simulink model "SHEV_EXAMPLE1"  (R2024a)
settings: Solver=VariableStepAuto  StartTime=0  StopTime=40  RelTol=1e-3
model workspace (MAT data in the model file):
  rpm0 = Simulink.Parameter
  rpm0.Value = 2000
  rpm0.Complexity = 'real'
  rpm0.Dimensions = [1 1]
  rpm0.DataType = 'double'
  v0 = Simulink.Parameter
  v0.Value = 15
  v0.Complexity = 'real'
  v0.Dimensions = [1 1]
  v0.DataType = 'double'
  wheel_radius = Simulink.Parameter
  wheel_radius.Value = 0.3
  wheel_radius.Complexity = 'real'
  wheel_radius.Dimensions = [1 1]
  wheel_radius.DataType = 'double'
libraries: fl_lib x27, nesl_utility x16, sdl_lib x8, autolibshared x2, ee_lib x1
settings Model: Creator=DELL  LastModifiedBy=DELL

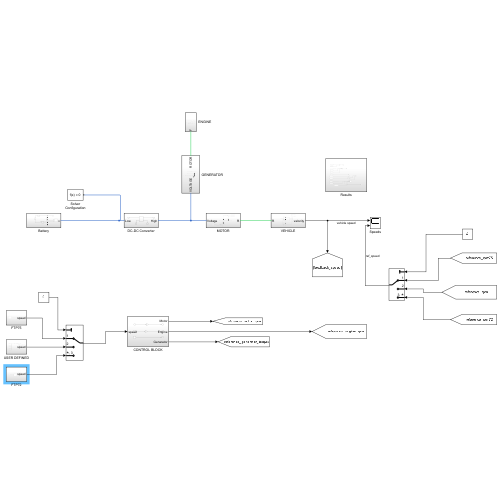
[thumbnail: Simulink's stored preview of the top-level diagram]
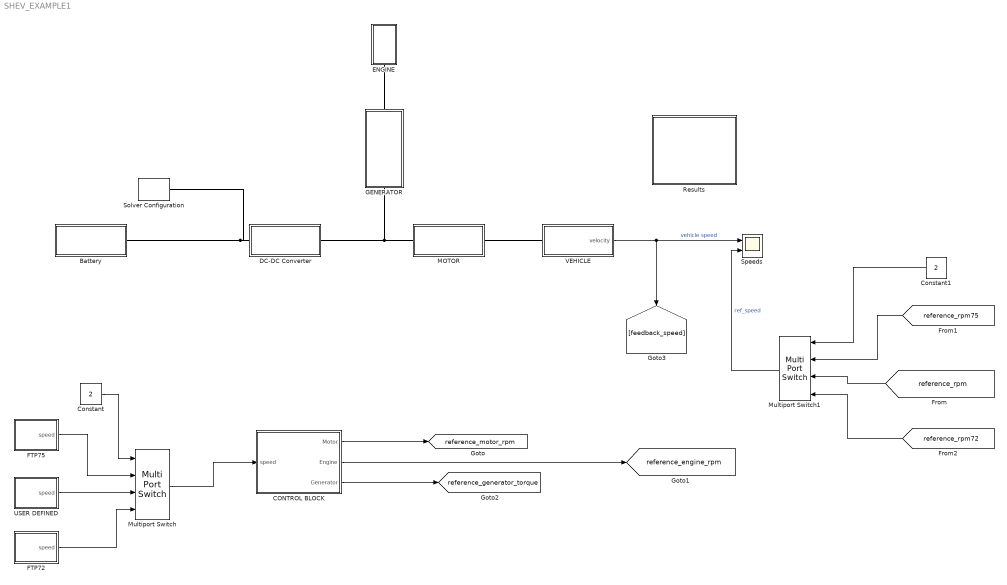
== system SHEV_EXAMPLE1 ==
  Battery : Subsystem
  CONTROL BLOCK : Subsystem
  Constant : Constant  Value=2
  Constant1 : Constant  Value=2
  DC-DC Converter : Subsystem
  ENGINE : Subsystem
  FTP72 : Subsystem
  FTP75 : Subsystem
  GENERATOR : Subsystem
  MOTOR : Subsystem
  Multiport Switch : MultiPortSwitch  SaturateOnIntegerOverflow=off  InputSameDT=off
  Multiport Switch1 : MultiPortSwitch  SaturateOnIntegerOverflow=off  InputSameDT=off
  Results : Subsystem
  Solver Configuration : nesl_utility/Solver Configuration  PhysicalDomain=network_engine_domain  SubClassName=solver  LeftPortType=input  RightPortType=generic  Tones=[]  Harmonics=[]  SimulateNoise=off  Profile=off  UseLocalSampling=off  EnableSwitchedLinearOptims=on  FrequencyDomain=off  UseCCode=off  RelTol=0.001  AbsTol=0.001  MinStep=1e-09  ToWorkspace=off  RevertToSquareIcSolve=off  NumHomotopyIterations=100  PhasorMode=off  PhasorModeNumHarmonics=1  ConsistencySolver=NEWTON_XTOL_AFTER_FTOL  IndexReductionMethod=DerivativeReplacement  DoDC=off  ResidualTolerance=1e-09  ConsistencyTolSource=GLOBAL  ConsistencyAbsTol=0.001  ConsistencyRelTol=0.001  ConsistencyTolFactor=0.001  UseLocalSolver=off  LocalSolverChoice=NE_BACKWARD_EULER_ADVANCER  ResolveIndetEquations=on  FunctionEvalNumThread=1  LocalSolverSampleTime=0.001  DoFixedCost=off  MaxNonlinIter=3  MaxModeIter=2  ComputeImpulses=off  ImpulseIterations=2  LinearAlgebra=auto  LinearAlgebraNumThread=0  EquationFormulation=NE_TIME_EF  DelaysMemoryBudget=1024  AutomaticFiltering=on  FilteringTimeConstant=0.001  PartitionStorageMethod=AS_NEEDED  PartitionMemoryBudget=1024  PartitionMethod=ROBUST  MultibodyUseLocalSolver=off  MultibodyLocalSolverChoice=ODE1  MultibodyLocalSolverSampleTime=0.001
  Speeds : Scope  NumInputPorts=2
  USER DEFINED : Subsystem
  VEHICLE : Subsystem
  tag scope: reference_engine_rpm=global, reference_generator_torque=global, reference_motor_rpm=global
  wires:
  [reference_rpm] -> Multiport Switch1/3
  CONTROL BLOCK/1(Motor) -> [reference_motor_rpm]
  VEHICLE/1(velocity) -> [feedback_speed], Speeds/1  "vehicle speed"
  CONTROL BLOCK/3(Generator) -> [reference_generator_torque]
  CONTROL BLOCK/2(Engine) -> [reference_engine_rpm]
  Constant/1 -> Multiport Switch/1
  FTP75/1(speed) -> Multiport Switch/2
  USER DEFINED/1(speed) -> Multiport Switch/3
  FTP72/1(speed) -> Multiport Switch/4
  Multiport Switch/1 -> CONTROL BLOCK/1(speed)
  Constant1/1 -> Multiport Switch1/1
  [reference_rpm75] -> Multiport Switch1/2
  [reference_rpm72] -> Multiport Switch1/4
  Multiport Switch1/1 -> Speeds/2  "ref_speed"
  connections:
  DC-DC Converter/LConn1 -- Solver Configuration/RConn1 -- Battery/RConn1
  MOTOR/RConn1 -- VEHICLE/LConn1
  ENGINE/LConn1 -- GENERATOR/RConn1
  DC-DC Converter/RConn1 -- GENERATOR/LConn1 -- MOTOR/LConn1

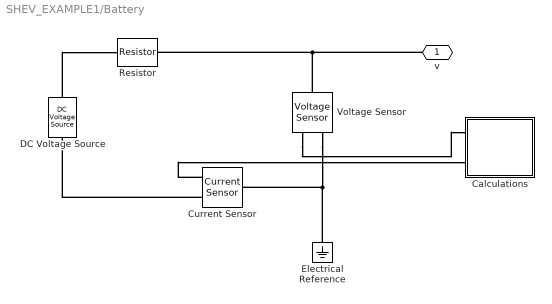
== system SHEV_EXAMPLE1/Battery ==
  Calculations : Subsystem
  Current Sensor : fl_lib/Electrical/Electrical Sensors/Current Sensor
  DC Voltage Source : ee_lib/Additional Components/SPICE Sources/DC Voltage Source  DC=200 V
  Electrical Reference : fl_lib/Electrical/Electrical Elements/Electrical Reference
  Resistor : fl_lib/Electrical/Electrical Elements/Resistor  R=0.05 Ohm  i_specify=off  i_priority=None  i=0 A  i_nominal_specify=off  i_nominal_value=1  i_nominal_unit=A  v_specify=off  v_priority=None  v=0 V  v_nominal_specify=off  v_nominal_value=1  v_nominal_unit=V
  Voltage Sensor : fl_lib/Electrical/Electrical Sensors/Voltage Sensor
  v : PMIOPort  Side=Right
  connections:
  DC Voltage Source/LConn1 -- Resistor/LConn1
  Current Sensor/RConn2 -- DC Voltage Source/RConn1
  Voltage Sensor/LConn1 -- Resistor/RConn1 -- v/RConn1
  Voltage Sensor/RConn2 -- Current Sensor/LConn1 -- Electrical Reference/LConn1
  Voltage Sensor/RConn1 -- Calculations/RConn1
  Current Sensor/RConn1 -- Calculations/RConn2

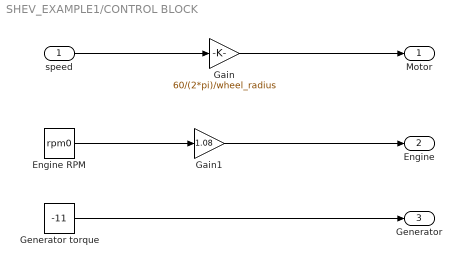
== system SHEV_EXAMPLE1/CONTROL BLOCK ==
  speed : Inport
  Engine RPM : Constant  Value=rpm0
  Gain : Gain  Gain=60/(2*pi)/wheel_radius
  Gain1 : Gain  Gain=1.08
  "Generator torque " : Constant  Value=-11
  Motor : Outport
  Engine : Outport  Port=2
  Generator : Outport  Port=3
  wires:
  speed/1 -> Gain/1
  Gain/1 -> Motor/1
  Engine RPM/1 -> Gain1/1
  Gain1/1 -> Engine/1
  "Generator torque "/1 -> Generator/1

== system SHEV_EXAMPLE1/DC-DC Converter ==
  Electrical Reference : fl_lib/Electrical/Electrical Elements/Electrical Reference
  Electrical Reference1 : fl_lib/Electrical/Electrical Elements/Electrical Reference
  Ideal Transformer : fl_lib/Electrical/Electrical Elements/Ideal Transformer  n=200/500  i1_specify=off  i1_priority=None  i1=0 A  i1_nominal_specify=off  i1_nominal_value=1  i1_nominal_unit=A  v1_specify=off  v1_priority=None  v1=0 V  v1_nominal_specify=off  v1_nominal_value=1  v1_nominal_unit=V  i2_specify=off  i2_priority=None  i2=0 A  i2_nominal_specify=off  i2_nominal_value=1  i2_nominal_unit=A  v2_specify=off  v2_priority=None  v2=0 V  v2_nominal_specify=off  v2_nominal_value=1  v2_nominal_unit=V
  Low : PMIOPort  Side=Left
  High : PMIOPort  Port=2  Side=Right
  connections:
  Ideal Transformer/LConn2 -- Electrical Reference/LConn1
  Ideal Transformer/RConn2 -- Electrical Reference1/LConn1
  Low/RConn1 -- Ideal Transformer/LConn1
  High/RConn1 -- Ideal Transformer/RConn1

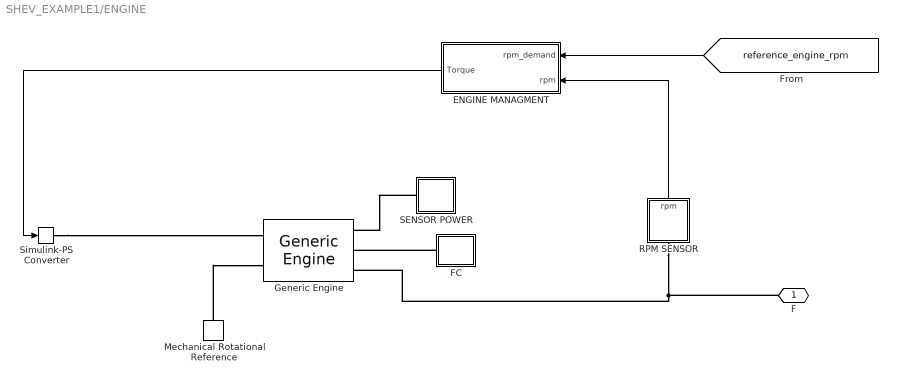
== system SHEV_EXAMPLE1/ENGINE ==
  ENGINE MANAGMENT : Subsystem
  FC : Subsystem
  Generic Engine : sdl_lib/Engines & Motors/Generic Engine  input_type=sdl.enum.GenericEngineInputType.NormalizedThrottle  model_parameterization=sdl.enum.engineParameterization.polynomial  engine_type=sdl.enum.engineType.SI  Trq_max=380 N*m  w_Trq_max=4300 rpm  P_max=50e3 W  w_P_max=5500 rpm  w_max=7000 rpm  w_min=500 rpm  w_tab=[500, 1000, 2000, 3000, 4300, 5000, 6000, 7000] rpm  trq_tab=[250, 280, 330, 360, 380, 370, 350, 310] N*m  pwr_tab=[10, 30, 70, 110, 165, 190, 220, 230] kW  interp_method=simscape.enum.interpolation.linear  w_thr=20 rpm  model_inertia=sdl.enum.model_inertia.on  inertia=0.2 kg*m^2  initial_velocity=rpm0 rpm  model_time_constant=sdl.enum.lagOffOn.on  time_constant=0.2 s  initial_normalized_throttle=0  fc_model=sdl.enum.fuel_consumption_model.BSFCSpeedBMEP  fc_per_rev=25 mg/rev  fc_w_tab=[ 1000 2e+3 3e+3 4e+3 5e+3 6e+3 ] rpm  fc_trq_tab=[0, 80, 160, 200, 240, 320, 360, 400] N*m  fc_tab=[.5, .9, 1.4, 1.6, 1.9, 2.7, 3.4, 4.4; 1, 1.7, 2.7, 3.1, 3.6, 5, 6, 7.4; 1.4, 2.7, 4, 4.8, 5.6, 7.5, 8.5, 10.5; 2, 3.6, 5.8, 6.7, 8, 10.4, 11.7, 13.3; 2.5, 4.8, 7.9, 9.4, 10.8, 14, 16.2, 18.6; 3.1, 6, 10.3, 11.9, 13.8, 18.4, 22, 26.5] g/s  bmep_tab=[ 0 250 500 625 750 1000 1.15e+3 1.25e+3 ] kPa  bsfc_tab=[ 410 380 300 280 270 290 320 380; 410 370 290 270 260 270 285 320; 415 380 290 275 265 270 270 300; 420 390 310 290 285 280 280 285; 430 410 340 320 310 300 310 320; 450 430 370 340 330 330 350 380 ] g/hr/kW  fc_interp_method=simscape.enum.interpolation.linear  displaced_volume=400 cm^3  rev_per_cycle=2  idle_speed=false  idle_speed_reference=1000 rpm  tau_controller=1 s  idle_w_thr=1 rpm  redline=false  redline_speed=5000 rpm  tau_redline=1 s  redline_w_thr=1 rpm
      settings: InternalSimscapePortConfiguration="{\"Bottom\":[],\"Left\":[{\"id\":\"ThrNorm\",\"label\":\"Thr\",\"type\":\"input\"},{\"id\":\"B\",\"label\":\"B\",\"type\":\"foundation.mechanical.rotational.rotational\"}],\"Right\":[{\"id\":\"P\",\"label\":\"P\",\"type\":\"output\"},{\"id\":\"FC\",\"label\":\"FC\",\"type\":\"output\"},{\"id\":\"F\",\"label\":\"F\",\"type\":\"foundation.mechanical.rotational.rotational\"}],\"Top\":[]}"
  Mechanical Rotational Reference : fl_lib/Mechanical/Rotational Elements/Mechanical Rotational Reference
  RPM SENSOR : Subsystem
  SENSOR POWER : Subsystem
  Simulink-PS Converter : nesl_utility/Simulink-PS Converter  PhysicalDomain=network_engine_domain  SubClassName=ps_input  LeftPortType=input  RightPortType=output  PseudoPeriodic=off  Frequencies=[]  NoiseDistribution=none  NoiseParameters=[]  Unit=1  AffineConversion=off  FilteringAndDerivatives=zero  SimscapeFilterOrder=1  InputFilterTimeConstant=0.001  UdotUserProvided=0
  F : PMIOPort  Side=Left
  wires:
  [reference_engine_rpm] -> ENGINE MANAGMENT/1(rpm_demand)
  RPM SENSOR/1(rpm) -> ENGINE MANAGMENT/2(rpm)
  ENGINE MANAGMENT/1(Torque) -> Simulink-PS Converter/1
  connections:
  Mechanical Rotational Reference/LConn1 -- Generic Engine/LConn2
  Simulink-PS Converter/RConn1 -- Generic Engine/LConn1
  SENSOR POWER/LConn1 -- Generic Engine/RConn1
  FC/LConn1 -- Generic Engine/RConn2
  RPM SENSOR/LConn1 -- F/RConn1 -- Generic Engine/RConn3

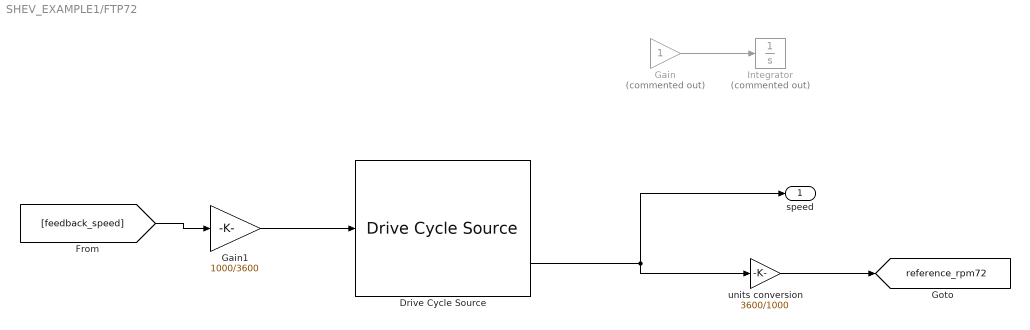
== system SHEV_EXAMPLE1/FTP72 ==
  Drive Cycle Source : autolibshared/Drive Cycle Source  cycleVar=FTP72  fileVar=cycleFTP75.mat  tfinal="1372  seconds"  cycleRepeat=off  outAccPort=off  outGearPort=off  gearList=No gear data  t_wot1=5  xdot_woto=0  xdot_wot1=30  t_wot2=20  xdot_wot2=0  t_wotend=30  srcUnit=m/s  outUnit=m/s  srcAccUnit=m/s/s  outAccUnit=m/s^2  dt=0  aMode=1  faultOption=on  velBnd=2  velBndUnit=mph  inUnit=m/s  timeBnd=1  failOption=off  stopSim=off  maxFaultCnt=10  maxFaultTime=2  maxTotFaultTime=15  traceOption=off  dtTrace=1  traceWindow=10  lastDCname=FTP72  lastOutUnit=mph  lastDT=0  lastTB=1  lastSB=2  forceCalcBound=off
  Gain : Gain  Commented=on
  Gain1 : Gain  Gain=1000/3600
  Integrator : Integrator  Commented=on  InitialCondition=v0
  units conversion : Gain  Gain=3600/1000
  speed : Outport
  tag scope: reference_rpm72=global
  wires:
  Gain/1 -> Integrator/1
  units conversion/1 -> [reference_rpm72]
  Drive Cycle Source/2 -> speed/1, units conversion/1
  Gain1/1 -> Drive Cycle Source/1
  [feedback_speed] -> Gain1/1

== system SHEV_EXAMPLE1/FTP75 ==
  Drive Cycle Source : autolibshared/Drive Cycle Source  cycleVar=FTP75  fileVar=cycleFTP75.mat  tfinal="2474  seconds"  cycleRepeat=off  outAccPort=off  outGearPort=off  gearList=No gear data  t_wot1=5  xdot_woto=0  xdot_wot1=30  t_wot2=20  xdot_wot2=0  t_wotend=30  srcUnit=m/s  outUnit=m/s  srcAccUnit=m/s/s  outAccUnit=m/s^2  dt=0  aMode=1  faultOption=off  velBnd=2  velBndUnit=mph  inUnit=m/s  timeBnd=1  failOption=off  stopSim=off  maxFaultCnt=10  maxFaultTime=2  maxTotFaultTime=15  traceOption=off  dtTrace=1  traceWindow=10  lastDCname=FTP75  lastOutUnit=mph  lastDT=0  lastTB=1  lastSB=2  forceCalcBound=off
  units conversion : Gain  Gain=3600/1000
  speed : Outport
  tag scope: reference_rpm75=global
  wires:
  units conversion/1 -> [reference_rpm75]
  Drive Cycle Source/1 -> units conversion/1, speed/1

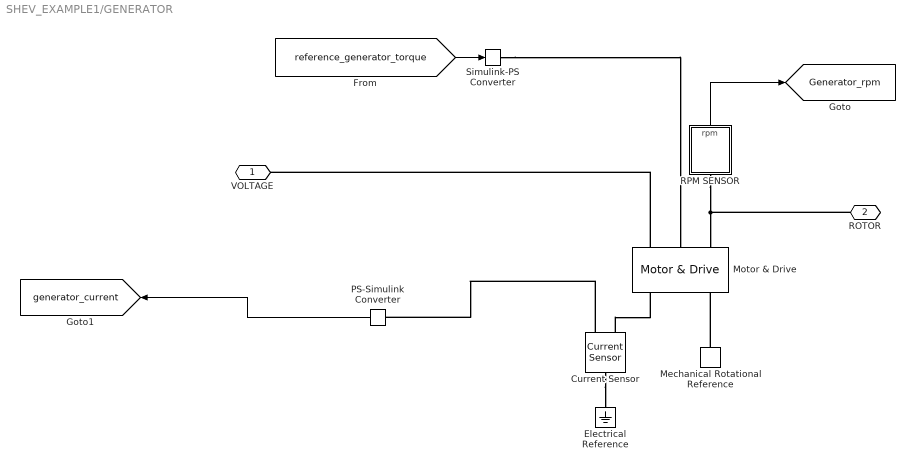
== system SHEV_EXAMPLE1/GENERATOR ==
  Current Sensor : fl_lib/Electrical/Electrical Sensors/Current Sensor
  Electrical Reference : fl_lib/Electrical/Electrical Elements/Electrical Reference
  Mechanical Rotational Reference : fl_lib/Mechanical/Rotational Elements/Mechanical Rotational Reference
  Motor & Drive : sdl_lib/Engines & Motors/Motor & Drive  torque_max=400 N*m  power_max=200 kW  Tc=0.2 s  eff=97  w_eff=600 rpm  T_eff=300 N*m  thermal_port=simscape.enum.thermaleffects.omit  thermal_mass=100 J/K  temperature_specify=off  temperature_priority=High  temperature=300 K  temperature_nominal_specify=off  temperature_nominal_value=1  temperature_nominal_unit=K
      settings: InternalSimscapePortConfiguration="{\"Bottom\":[],\"Left\":[{\"id\":\"Vp\",\"label\":\"+\",\"type\":\"foundation.electrical.electrical\"},{\"id\":\"Tr\",\"label\":\"Tr\",\"type\":\"input\"},{\"id\":\"R\",\"label\":\"R\",\"type\":\"foundation.mechanical.rotational.rotational\"}],\"Right\":[{\"id\":\"Vm\",\"label\":\"-\",\"type\":\"foundation.electrical.electrical\"},{\"id\":\"Omega\",\"label\":\"w\",\"type\":\"output\"},{\"id\":\"C\",\"label\":\"C\",\"type\":\"foundation.mechanical.rotational.rotational\"}],\"Top\":[]}"
  PS-Simulink Converter : nesl_utility/PS-Simulink Converter  PhysicalDomain=network_engine_domain  SubClassName=ps_output  LeftPortType=input  RightPortType=output  PseudoPeriodic=off  Frequencies=[]  VectorFormat=1-D array  Unit=A  AffineConversion=off
  RPM SENSOR : Subsystem
  Simulink-PS Converter : nesl_utility/Simulink-PS Converter  PhysicalDomain=network_engine_domain  SubClassName=ps_input  LeftPortType=input  RightPortType=output  PseudoPeriodic=off  Frequencies=[]  NoiseDistribution=none  NoiseParameters=[]  Unit=N*m  AffineConversion=off  FilteringAndDerivatives=zero  SimscapeFilterOrder=1  InputFilterTimeConstant=0.001  UdotUserProvided=0
  VOLTAGE : PMIOPort  Side=Left
  ROTOR : PMIOPort  Port=2  Side=Right
  tag scope: Generator_rpm=global, generator_current=global
  wires:
  [reference_generator_torque] -> Simulink-PS Converter/1
  RPM SENSOR/1(rpm) -> [Generator_rpm]
  PS-Simulink Converter/1 -> [generator_current]
  connections:
  RPM SENSOR/LConn1 -- Motor & Drive/LConn3 -- ROTOR/RConn1
  Simulink-PS Converter/RConn1 -- Motor & Drive/LConn2
  Mechanical Rotational Reference/LConn1 -- Motor & Drive/RConn3
  Current Sensor/RConn1 -- PS-Simulink Converter/LConn1
  Motor & Drive/LConn1 -- VOLTAGE/RConn1
  Current Sensor/LConn1 -- Electrical Reference/LConn1
  Current Sensor/RConn2 -- Motor & Drive/RConn1

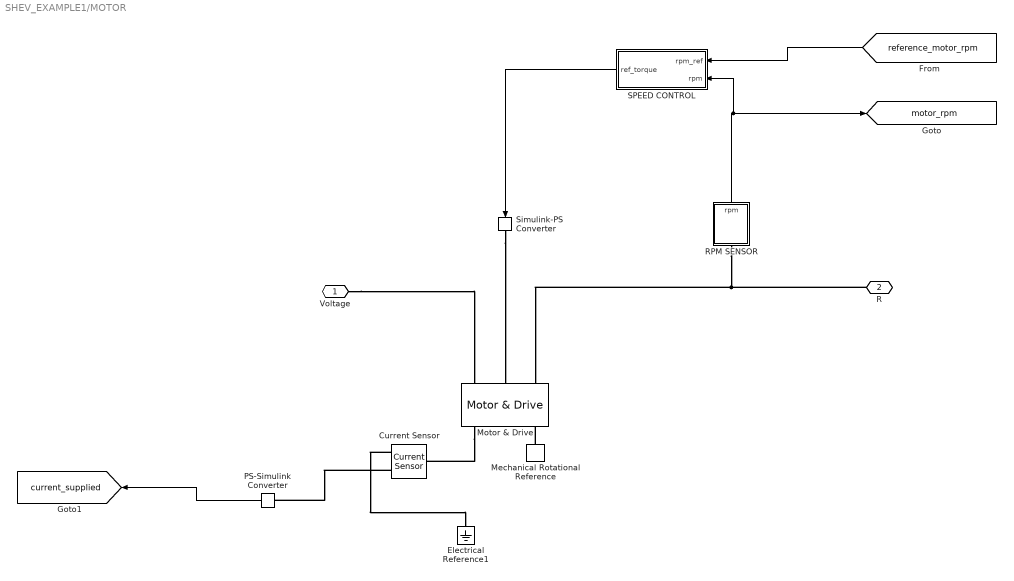
== system SHEV_EXAMPLE1/MOTOR ==
  Current Sensor : fl_lib/Electrical/Electrical Sensors/Current Sensor
  Electrical Reference1 : fl_lib/Electrical/Electrical Elements/Electrical Reference
  Mechanical Rotational Reference : fl_lib/Mechanical/Rotational Elements/Mechanical Rotational Reference
  Motor & Drive : sdl_lib/Engines & Motors/Motor & Drive  torque_max=400 N*m  power_max=200 kW  Tc=0.2 s  eff=97  w_eff=600 rpm  T_eff=300 N*m  thermal_port=simscape.enum.thermaleffects.omit  thermal_mass=100 J/K  temperature_specify=off  temperature_priority=High  temperature=300 K  temperature_nominal_specify=off  temperature_nominal_value=1  temperature_nominal_unit=K
      settings: InternalSimscapePortConfiguration="{\"Bottom\":[],\"Left\":[{\"id\":\"Vp\",\"label\":\"+\",\"type\":\"foundation.electrical.electrical\"},{\"id\":\"Tr\",\"label\":\"Tr\",\"type\":\"input\"},{\"id\":\"R\",\"label\":\"R\",\"type\":\"foundation.mechanical.rotational.rotational\"}],\"Right\":[{\"id\":\"Vm\",\"label\":\"-\",\"type\":\"foundation.electrical.electrical\"},{\"id\":\"Omega\",\"label\":\"w\",\"type\":\"output\"},{\"id\":\"C\",\"label\":\"C\",\"type\":\"foundation.mechanical.rotational.rotational\"}],\"Top\":[]}"
  PS-Simulink Converter : nesl_utility/PS-Simulink Converter  PhysicalDomain=network_engine_domain  SubClassName=ps_output  LeftPortType=input  RightPortType=output  PseudoPeriodic=off  Frequencies=[]  VectorFormat=1-D array  Unit=A  AffineConversion=off
  RPM SENSOR : Subsystem
  SPEED CONTROL : Subsystem
  Simulink-PS Converter : nesl_utility/Simulink-PS Converter  PhysicalDomain=network_engine_domain  SubClassName=ps_input  LeftPortType=input  RightPortType=output  PseudoPeriodic=off  Frequencies=[]  NoiseDistribution=none  NoiseParameters=[]  Unit=N*m  AffineConversion=off  FilteringAndDerivatives=zero  SimscapeFilterOrder=1  InputFilterTimeConstant=0.001  UdotUserProvided=0
  Voltage : PMIOPort  Side=Left
  R : PMIOPort  Port=2  Side=Right
  tag scope: current_supplied=global, motor_rpm=global
  wires:
  RPM SENSOR/1(rpm) -> SPEED CONTROL/2(rpm), [motor_rpm]
  SPEED CONTROL/1(ref_torque) -> Simulink-PS Converter/1
  [reference_motor_rpm] -> SPEED CONTROL/1(rpm_ref)
  PS-Simulink Converter/1 -> [current_supplied]
  connections:
  Voltage/RConn1 -- Motor & Drive/LConn1
  Mechanical Rotational Reference/LConn1 -- Motor & Drive/RConn3
  R/RConn1 -- RPM SENSOR/LConn1 -- Motor & Drive/LConn3
  Simulink-PS Converter/RConn1 -- Motor & Drive/LConn2
  Current Sensor/RConn1 -- PS-Simulink Converter/LConn1
  Motor & Drive/RConn1 -- Current Sensor/LConn1
  Current Sensor/RConn2 -- Electrical Reference1/LConn1

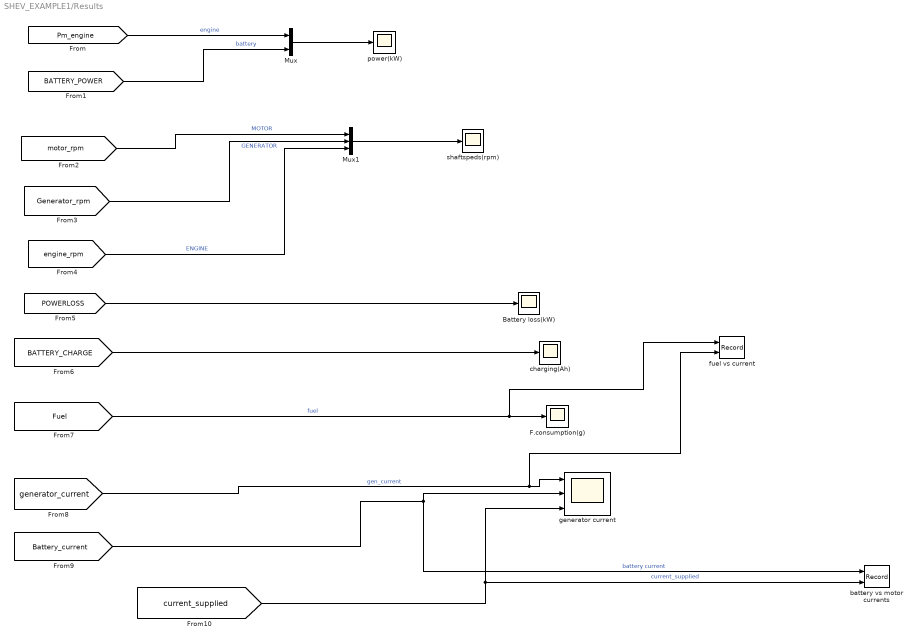
== system SHEV_EXAMPLE1/Results ==
  Battery loss(kW) : Scope
  F.consumption(g) : Scope
  Mux : Mux  Inputs=2
  Mux1 : Mux  Inputs=3
  battery vs motor currents : Record  FileSettingsInternal="{\"entries\":[{\"content\":{\"excelSettings\":{\"content\":{},\"type\":\"Streamout.ExcelSettings\"}},\"type\":\"Streamout.FileSettingStorage\",\"uuid\":\"\"}],\"packageUris\":[\"http:\\/\\/schema.mathworks.com\\/mf0\\/streamout_blocks\\/R2020a\"],\"version\":\"1.0\"}"  Layout=[1 1]  SignalsInternal="{\"entries\":[{\"content\":{\"signals\":[{\"content\":{\"blockPath\":[],\"dimensions\":[1],\"domain\":\"\",\"lineColor\":\"#0072bd\",\"lineWidth\":2,\"port\":1,\"sid\":[\"\"],\"signalID\":1,\"signalName\":\"battery current\"},\"type\":\"RecordBlkView.Signal\",\"uuid\":\"\"},{\"content\":{\"blockPath\":[],\"dimensions\":[1],\"domain\":\"\",\"lineColor\":\"#139fff\",\"plots\":[ 1 ],\"port\":2,\"sid\":[\"\"],\"signalID\":2,\"signalName\":\"current_supplied\"},\"type\":\"RecordBlkView.Signal\",\"uuid\":\"\"}]},\"type\":\"RecordBlkView.InputSignals\",\"uuid\":\"\"}],\"packageUris\":[\"http:\\/\\/schema.mathworks.com\\/mf0\\/streamout_blocks\\/R2020a\"],\"version\":\"1.0\"}"  VisualizationBindings="{\"xyplotplugin\":{\"info\":[{\"series\":[{\"bindingParametersList\":[{\"parameter\":\"Y-Axis\",\"signalID\":2,\"signalName\":\"current_supplied\"}],\"seriesID\":0}],\"subplotID\":1}]}}"  CompatibilityTag=XY
  charging(Ah) : Scope
  "fuel vs current " : Record  FileSettingsInternal="{\"entries\":[{\"content\":{\"excelSettings\":{\"content\":{},\"type\":\"Streamout.ExcelSettings\"}},\"type\":\"Streamout.FileSettingStorage\",\"uuid\":\"\"}],\"packageUris\":[\"http:\\/\\/schema.mathworks.com\\/mf0\\/streamout_blocks\\/R2020a\"],\"version\":\"1.0\"}"  Layout=[1 1]  SignalsInternal="{\"entries\":[{\"content\":{\"signals\":[{\"content\":{\"blockPath\":[],\"dimensions\":[1],\"domain\":\"\",\"lineColor\":\"#edb120\",\"lineWidth\":2,\"port\":1,\"sid\":[\"\"],\"signalID\":1,\"signalName\":\"fuel\"},\"type\":\"RecordBlkView.Signal\",\"uuid\":\"\"},{\"content\":{\"blockPath\":[],\"dimensions\":[1],\"domain\":\"\",\"lineColor\":\"#7e2f8e\",\"lineWidth\":2,\"port\":2,\"sid\":[\"\"],\"signalID\":2,\"signalName\":\"gen_current\"},\"type\":\"RecordBlkView.Signal\",\"uuid\":\"\"}]},\"type\":\"RecordBlkView.InputSignals\",\"uuid\":\"\"}],\"packageUris\":[\"http:\\/\\/schema.mathworks.com\\/mf0\\/streamout_blocks\\/R2020a\"],\"version\":\"1.0\"}"  VisualizationBindings="{\"xyplotplugin\":{\"info\":[{\"series\":[],\"subplotID\":1}]}}"  CompatibilityTag=XY
  generator current : Scope  NumInputPorts=3
  power(kW) : Scope
  shaftspeds(rpm) : Scope
  wires:
  Mux/1 -> power(kW)/1
  [Pm_engine] -> Mux/1  "engine"
  [BATTERY_POWER] -> Mux/2  "battery"
  [motor_rpm] -> Mux1/1  "MOTOR"
  [Generator_rpm] -> Mux1/2  "GENERATOR"
  [engine_rpm] -> Mux1/3  "ENGINE"
  [POWERLOSS] -> Battery loss(kW)/1
  [BATTERY_CHARGE] -> charging(Ah)/1
  [Fuel] -> "fuel vs current "/1, F.consumption(g)/1  "fuel"
  Mux1/1 -> shaftspeds(rpm)/1
  [generator_current] -> "fuel vs current "/2, generator current/1  "gen_current"
  [Battery_current] -> battery vs motor currents/1, generator current/2  "battery current"
  [current_supplied] -> generator current/3, battery vs motor currents/2  "current_supplied"

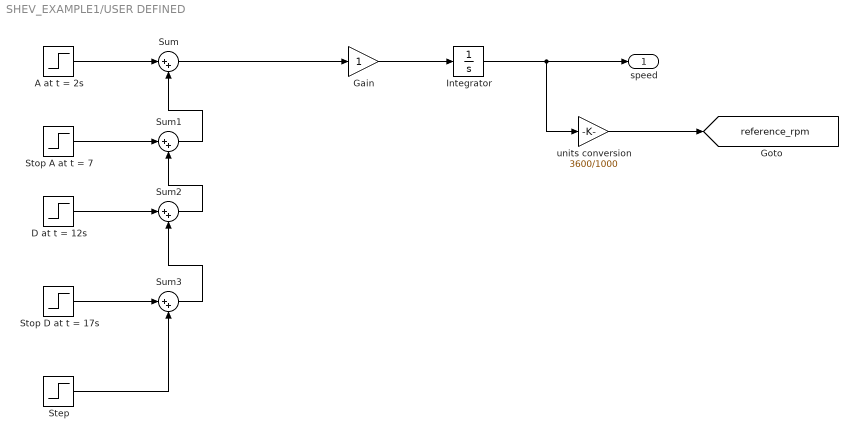
== system SHEV_EXAMPLE1/USER DEFINED ==
  A at t = 2s : Step  Time=2  SampleTime=0
  D at t = 12s : Step  Time=12  After=-1  SampleTime=0
  Gain : Gain
  Integrator : Integrator  InitialCondition=v0
  Step : Step  Time=36  SampleTime=0
  Stop A at t = 7 : Step  Time=7  After=-1  SampleTime=0
  Stop D at t = 17s : Step  Time=17  SampleTime=0
  Sum{,1..3} (4 alike) : Sum  Inputs=|++
  units conversion : Gain  Gain=3600/1000
  speed : Outport
  tag scope: reference_rpm=global
  wires:
  units conversion/1 -> [reference_rpm]
  Gain/1 -> Integrator/1
  Integrator/1 -> units conversion/1, speed/1
  Sum3/1 -> Sum2/2
  Sum2/1 -> Sum1/2
  Stop D at t = 17s/1 -> Sum3/1
  Step/1 -> Sum3/2
  Sum1/1 -> Sum/2
  Sum/1 -> Gain/1
  A at t = 2s/1 -> Sum/1
  Stop A at t = 7/1 -> Sum1/1
  D at t = 12s/1 -> Sum2/1

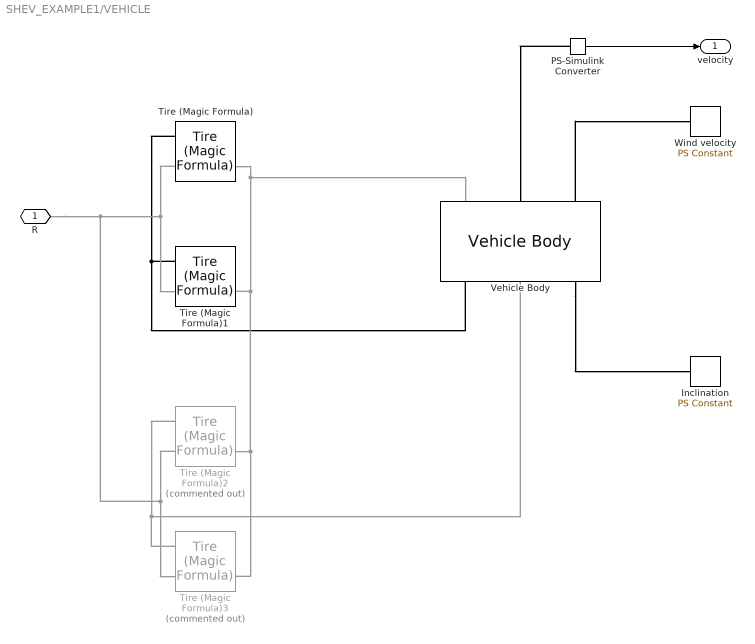
== system SHEV_EXAMPLE1/VEHICLE ==
  Inclination : fl_lib/Physical Signals/Sources/PS Constant  constant=0
  PS-Simulink Converter : nesl_utility/PS-Simulink Converter  PhysicalDomain=network_engine_domain  SubClassName=ps_output  LeftPortType=input  RightPortType=output  PseudoPeriodic=off  Frequencies=[]  VectorFormat=1-D array  Unit=km/hr  AffineConversion=off
  Tire (Magic Formula) : sdl_lib/Tires & Vehicles/Tire (Magic Formula)  parameterization=sdl.enum.magic_tire_model.peak  F_z1=3000 N  F_x1=3500 N  kappa1=10  B_m=10  C_m=1.9  D_m=1  E_m=0.97  fz0=4000 N  p_Cx=1.685  p_Dx=[1.21, -.037]  p_Ex=[.344, .095, -.02, 0]  p_Kx=[21.51, -.163, .245]  p_Hx=[-.002, .002]  p_Vx=[0, 0]  rolling_radius_model=sdl.enum.RollingRadiusParameterization.Constant  r_e=wheel_radius m  r_0=0.3 m  breff=8.39  dreff=0.26  freff=0.074  q_re0=0.99  q_v1=0.008  longvl=17 m/s  cz=5e5 N/m  model_resistance=false  resistance_model=sdl.enum.rollingResistanceParameterization.constant  coeff=0.015  p_tire=250e3 Pa  alpha=-0.003  beta=0.97  coeff_a=84e-4  coeff_b=6.2e-4 s/m  coeff_c=1.6e-4 s^2/m^2  p_tire0=240e3 Pa  fz0_resistance=4000 N  vH0=16 m/s  q_Sy=[.0082, 0, .0014, .001, 0, 0, 1.08, -.5]  v_thr=0.001 m/s  enable_scaling_coefficients=false  lfzO=1  lcx=1  lmux=1  lex=1  lkx=1  lhx=1  lvx=1  lmy=1  model_compliance=sdl.enum.compliance.off  stiffness=1e6 N/m  damping=1000 N*s/m  model_inertia=sdl.enum.model_inertia.on  inertia=1e-2 kg*m^2  initial_velocity=v0/wheel_radius rad/s  vxlow=1 m/s  v_tr_thr=(0.1)*(0.1) m/s  kpumin=-1e5  kpumax=1e5
  Tire (Magic Formula)1 : sdl_lib/Tires & Vehicles/Tire (Magic Formula)  parameterization=sdl.enum.magic_tire_model.peak  F_z1=3000 N  F_x1=3500 N  kappa1=10  B_m=10  C_m=1.9  D_m=1  E_m=0.97  fz0=4000 N  p_Cx=1.685  p_Dx=[1.21, -.037]  p_Ex=[.344, .095, -.02, 0]  p_Kx=[21.51, -.163, .245]  p_Hx=[-.002, .002]  p_Vx=[0, 0]  rolling_radius_model=sdl.enum.RollingRadiusParameterization.Constant  r_e=wheel_radius m  r_0=0.3 m  breff=8.39  dreff=0.26  freff=0.074  q_re0=0.99  q_v1=0.008  longvl=17 m/s  cz=5e5 N/m  model_resistance=false  resistance_model=sdl.enum.rollingResistanceParameterization.constant  coeff=0.015  p_tire=250e3 Pa  alpha=-0.003  beta=0.97  coeff_a=84e-4  coeff_b=6.2e-4 s/m  coeff_c=1.6e-4 s^2/m^2  p_tire0=240e3 Pa  fz0_resistance=4000 N  vH0=16 m/s  q_Sy=[.0082, 0, .0014, .001, 0, 0, 1.08, -.5]  v_thr=0.001 m/s  enable_scaling_coefficients=false  lfzO=1  lcx=1  lmux=1  lex=1  lkx=1  lhx=1  lvx=1  lmy=1  model_compliance=sdl.enum.compliance.off  stiffness=1e6 N/m  damping=1000 N*s/m  model_inertia=sdl.enum.model_inertia.on  inertia=1e-2 kg*m^2  initial_velocity=v0/wheel_radius rad/s  vxlow=1 m/s  v_tr_thr=(0.1)*(0.1) m/s  kpumin=-1e5  kpumax=1e5
  Tire (Magic Formula)2 : sdl_lib/Tires & Vehicles/Tire (Magic Formula)  Commented=on  parameterization=sdl.enum.magic_tire_model.peak  F_z1=3000 N  F_x1=3500 N  kappa1=10  B_m=10  C_m=1.9  D_m=1  E_m=0.97  fz0=4000 N  p_Cx=1.685  p_Dx=[1.21, -.037]  p_Ex=[.344, .095, -.02, 0]  p_Kx=[21.51, -.163, .245]  p_Hx=[-.002, .002]  p_Vx=[0, 0]  rolling_radius_model=sdl.enum.RollingRadiusParameterization.Constant  r_e=wheel_radius m  r_0=0.3 m  breff=8.39  dreff=0.26  freff=0.074  q_re0=0.99  q_v1=0.008  longvl=17 m/s  cz=5e5 N/m  model_resistance=false  resistance_model=sdl.enum.rollingResistanceParameterization.constant  coeff=0.015  p_tire=250e3 Pa  alpha=-0.003  beta=0.97  coeff_a=84e-4  coeff_b=6.2e-4 s/m  coeff_c=1.6e-4 s^2/m^2  p_tire0=240e3 Pa  fz0_resistance=4000 N  vH0=16 m/s  q_Sy=[.0082, 0, .0014, .001, 0, 0, 1.08, -.5]  v_thr=0.001 m/s  enable_scaling_coefficients=false  lfzO=1  lcx=1  lmux=1  lex=1  lkx=1  lhx=1  lvx=1  lmy=1  model_compliance=sdl.enum.compliance.off  stiffness=1e6 N/m  damping=1000 N*s/m  model_inertia=sdl.enum.model_inertia.on  inertia=1e-2 kg*m^2  initial_velocity=v0/wheel_radius rad/s  vxlow=1 m/s  v_tr_thr=(0.1)*(0.1) m/s  kpumin=-1e5  kpumax=1e5
  Tire (Magic Formula)3 : sdl_lib/Tires & Vehicles/Tire (Magic Formula)  Commented=on  parameterization=sdl.enum.magic_tire_model.peak  F_z1=3000 N  F_x1=3500 N  kappa1=10  B_m=10  C_m=1.9  D_m=1  E_m=0.97  fz0=4000 N  p_Cx=1.685  p_Dx=[1.21, -.037]  p_Ex=[.344, .095, -.02, 0]  p_Kx=[21.51, -.163, .245]  p_Hx=[-.002, .002]  p_Vx=[0, 0]  rolling_radius_model=sdl.enum.RollingRadiusParameterization.Constant  r_e=wheel_radius m  r_0=0.3 m  breff=8.39  dreff=0.26  freff=0.074  q_re0=0.99  q_v1=0.008  longvl=17 m/s  cz=5e5 N/m  model_resistance=false  resistance_model=sdl.enum.rollingResistanceParameterization.constant  coeff=0.015  p_tire=250e3 Pa  alpha=-0.003  beta=0.97  coeff_a=84e-4  coeff_b=6.2e-4 s/m  coeff_c=1.6e-4 s^2/m^2  p_tire0=240e3 Pa  fz0_resistance=4000 N  vH0=16 m/s  q_Sy=[.0082, 0, .0014, .001, 0, 0, 1.08, -.5]  v_thr=0.001 m/s  enable_scaling_coefficients=false  lfzO=1  lcx=1  lmux=1  lex=1  lkx=1  lhx=1  lvx=1  lmy=1  model_compliance=sdl.enum.compliance.off  stiffness=1e6 N/m  damping=1000 N*s/m  model_inertia=sdl.enum.model_inertia.on  inertia=1e-2 kg*m^2  initial_velocity=v0/wheel_radius rad/s  vxlow=1 m/s  v_tr_thr=(0.1)*(0.1) m/s  kpumin=-1e5  kpumax=1e5
  Vehicle Body : sdl_lib/Tires & Vehicles/Vehicle Body  mass=1200 kg  n_w=2  x_f=1.4 m  x_r=1.6 m  y_c=0.5 m  mass_var=simscape.enum.onoff.off  g=9.81 m/s^2  liftoff_warning=simscape.enum.onoff.off  area=3 m^2  Cd=0.4  rho=1.18 kg/m^3  model_pitch=simscape.enum.onoff.off  inertia=4000 kg*m^2  suspension_model=sdl.enum.linearTLU.linear  k_f=1e4 N/m  b_f=1e4 N*s/m  k_r=1e4 N/m  b_r=1e4 N*s/m  k_f_TLU=[-2000, -1000, 0, 1000, 2000] N  x_f_TLU=[-.4, -.2, 0, .2, .4] m  b_f_TLU=[-200, -100, 0, 100, 200] N  v_f_TLU=[-4, -2, 0, 2, 4] m/s  k_r_TLU=[-2000, -1000, 0, 1000, 2000] N  x_r_TLU=[-.4, -.2, 0, .2, .4] m  b_r_TLU=[-200, -100, 0, 100, 200] N  v_r_TLU=[-4, -2, 0, 2, 4] m/s  interp_method=simscape.enum.interpolation.linear  extrap_method=simscape.enum.extrapolation.linear  model_hardstop=simscape.enum.onoff.off  upper_bound_f=.25 m  lower_bound_f=-.25 m  stop_k_f=1e6 N/m  stop_b_f=150 N*s/m  upper_bound_r=.25 m  lower_bound_r=-.25 m  stop_k_r=1e6 N/m  stop_b_r=150 N*s/m  initial_pitch=0 rad  initial_pitch_rate=0 rad/s  v_specify=on  v_priority=High  v=v0 m/s  v_nominal_specify=off  v_nominal_value=1  v_nominal_unit=m/s
  Wind velocity : fl_lib/Physical Signals/Sources/PS Constant  constant=0
  R : PMIOPort  Side=Left
  velocity : Outport
  wires:
  PS-Simulink Converter/1 -> velocity/1
  connections:
  PS-Simulink Converter/LConn1 -- Vehicle Body/LConn2
  Vehicle Body/LConn3 -- Wind velocity/RConn1
  Vehicle Body/RConn3 -- Inclination/RConn1
  Tire (Magic Formula)/LConn1 -- Tire (Magic Formula)1/LConn1 -- Vehicle Body/RConn1
  Tire (Magic Formula)2/LConn2 -- Tire (Magic Formula)/LConn2 -- Tire (Magic Formula)1/LConn2 -- R/RConn1 -- Tire (Magic Formula)3/LConn2
  Tire (Magic Formula)2/RConn2 -- Tire (Magic Formula)3/RConn2 -- Tire (Magic Formula)/RConn2 -- Vehicle Body/LConn1 -- Tire (Magic Formula)1/RConn2
  Tire (Magic Formula)2/LConn1 -- Tire (Magic Formula)3/LConn1 -- Vehicle Body/RConn2

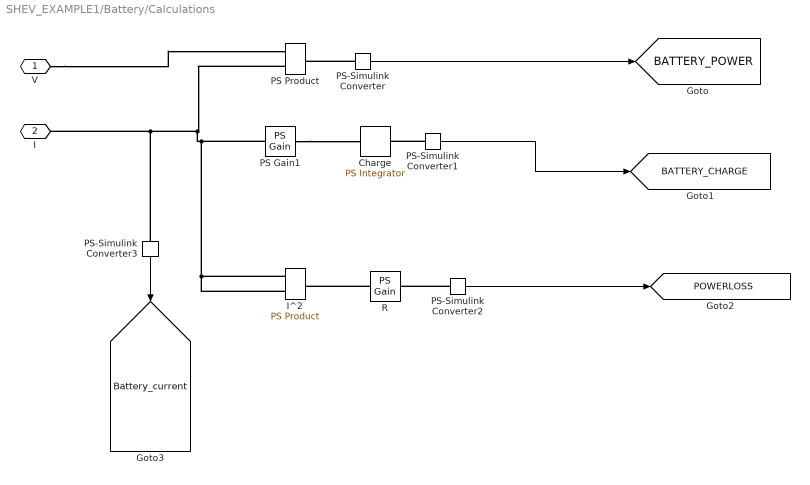
== system SHEV_EXAMPLE1/Battery/Calculations ==
  Charge : fl_lib/Physical Signals/Linear Operators/PS Integrator  reset_method=foundation.enum.IntegratorResetSpec.None  initial_condition_spec=foundation.enum.IntegratorICSpec.Internal  saturation_spec=foundation.enum.IntegratorSaturationSpec.None  saturation_source_spec=foundation.enum.IntegratorSaturationSourceSpec.Internal  x0=150 A*hr  xu=inf s  xl=-inf s
  I^2 : fl_lib/Physical Signals/Functions/PS Product
  PS Gain1 : fl_lib/Physical Signals/Functions/PS Gain  gain=-1
  PS Product : fl_lib/Physical Signals/Functions/PS Product
  PS-Simulink Converter : nesl_utility/PS-Simulink Converter  PhysicalDomain=network_engine_domain  SubClassName=ps_output  LeftPortType=input  RightPortType=output  PseudoPeriodic=off  Frequencies=[]  VectorFormat=1-D array  Unit=kW  AffineConversion=off
  PS-Simulink Converter1 : nesl_utility/PS-Simulink Converter  PhysicalDomain=network_engine_domain  SubClassName=ps_output  LeftPortType=input  RightPortType=output  PseudoPeriodic=off  Frequencies=[]  VectorFormat=1-D array  Unit=A*hr  AffineConversion=off
  PS-Simulink Converter2 : nesl_utility/PS-Simulink Converter  PhysicalDomain=network_engine_domain  SubClassName=ps_output  LeftPortType=input  RightPortType=output  PseudoPeriodic=off  Frequencies=[]  VectorFormat=inherit  Unit=inherit  AffineConversion=off
  PS-Simulink Converter3 : nesl_utility/PS-Simulink Converter  PhysicalDomain=network_engine_domain  SubClassName=ps_output  LeftPortType=input  RightPortType=output  PseudoPeriodic=off  Frequencies=[]  VectorFormat=1-D array  Unit=A  AffineConversion=off
  R : fl_lib/Physical Signals/Functions/PS Gain  gain=0.05 V/A
  V : PMIOPort  Side=Right
  I : PMIOPort  Port=2  Side=Right
  tag scope: BATTERY_CHARGE=global, BATTERY_POWER=global, Battery_current=global, POWERLOSS=global
  wires:
  PS-Simulink Converter/1 -> [BATTERY_POWER]
  PS-Simulink Converter1/1 -> [BATTERY_CHARGE]
  PS-Simulink Converter2/1 -> [POWERLOSS]
  PS-Simulink Converter3/1 -> [Battery_current]
  connections:
  R/LConn1 -- I^2/RConn1
  PS-Simulink Converter/LConn1 -- PS Product/RConn1
  V/RConn1 -- PS Product/LConn1
  PS Product/LConn2 -- I^2/LConn2 -- I^2/LConn1 -- PS Gain1/LConn1 -- PS-Simulink Converter3/LConn1 -- I/RConn1
  PS-Simulink Converter1/LConn1 -- Charge/RConn1
  PS Gain1/RConn1 -- Charge/LConn1
  PS-Simulink Converter2/LConn1 -- R/RConn1

== system SHEV_EXAMPLE1/ENGINE/ENGINE MANAGMENT ==
  rpm_demand : Inport
  rpm : Inport  Port=2
  Kp : Gain  Gain=1e-3  SaturateOnIntegerOverflow=on  OutDataTypeStr=Inherit: Same as input  ParamDataTypeStr=Inherit: Same as input
  Saturation : Saturate  UpperLimit=1  LowerLimit=0
  Sum : Sum  Inputs=+-
  Torque : Outport
  wires:
  rpm_demand/1 -> Sum/1
  rpm/1 -> Sum/2
  Sum/1 -> Kp/1
  Kp/1 -> Saturation/1
  Saturation/1 -> Torque/1

== system SHEV_EXAMPLE1/ENGINE/FC ==
  Integrator : Integrator
  PS-Simulink Converter : nesl_utility/PS-Simulink Converter  PhysicalDomain=network_engine_domain  SubClassName=ps_output  LeftPortType=input  RightPortType=output  PseudoPeriodic=off  Frequencies=[]  VectorFormat=1-D array  Unit=g/s  AffineConversion=off
  FC : PMIOPort  Side=Left
  tag scope: Fuel=global
  wires:
  PS-Simulink Converter/1 -> Integrator/1
  Integrator/1 -> [Fuel]
  connections:
  PS-Simulink Converter/LConn1 -- FC/RConn1

== system SHEV_EXAMPLE1/ENGINE/RPM SENSOR ==
  Ideal Rotational Motion Sensor : fl_lib/Mechanical/Mechanical Sensors/Ideal Rotational Motion Sensor  reference=foundation.enum.MeasurementReference.difference  acceleration_port=false  velocity_port=true  position_port=true  wrap_angle=false  offset=0 rad
  Mechanical Rotational Reference : fl_lib/Mechanical/Rotational Elements/Mechanical Rotational Reference
  PS-Simulink Converter : nesl_utility/PS-Simulink Converter  PhysicalDomain=network_engine_domain  SubClassName=ps_output  LeftPortType=input  RightPortType=output  PseudoPeriodic=off  Frequencies=[]  VectorFormat=1-D array  Unit=rpm  AffineConversion=off
  Sensor : TransferFcn  Denominator=[0.01 1]
  F : PMIOPort  Side=Left
  rpm : Outport
  tag scope: engine_rpm=global
  wires:
  PS-Simulink Converter/1 -> [engine_rpm], Sensor/1
  Sensor/1 -> rpm/1
  connections:
  F/RConn1 -- Ideal Rotational Motion Sensor/LConn1
  Mechanical Rotational Reference/LConn1 -- Ideal Rotational Motion Sensor/RConn1
  PS-Simulink Converter/LConn1 -- Ideal Rotational Motion Sensor/RConn2

== system SHEV_EXAMPLE1/ENGINE/SENSOR POWER ==
  PS-Simulink Converter : nesl_utility/PS-Simulink Converter  PhysicalDomain=network_engine_domain  SubClassName=ps_output  LeftPortType=input  RightPortType=output  PseudoPeriodic=off  Frequencies=[]  VectorFormat=1-D array  Unit=kW  AffineConversion=off
  P : PMIOPort  Side=Left
  tag scope: Pm_engine=global
  wires:
  PS-Simulink Converter/1 -> [Pm_engine]
  connections:
  PS-Simulink Converter/LConn1 -- P/RConn1

== system SHEV_EXAMPLE1/GENERATOR/RPM SENSOR ==
  Ideal Rotational Motion Sensor : fl_lib/Mechanical/Mechanical Sensors/Ideal Rotational Motion Sensor  reference=foundation.enum.MeasurementReference.difference  acceleration_port=false  velocity_port=true  position_port=true  wrap_angle=false  offset=0 rad
  Mechanical Rotational Reference : fl_lib/Mechanical/Rotational Elements/Mechanical Rotational Reference
  PS-Simulink Converter : nesl_utility/PS-Simulink Converter  PhysicalDomain=network_engine_domain  SubClassName=ps_output  LeftPortType=input  RightPortType=output  PseudoPeriodic=off  Frequencies=[]  VectorFormat=1-D array  Unit=rpm  AffineConversion=off
  R : PMIOPort  Side=Left
  rpm : Outport
  wires:
  PS-Simulink Converter/1 -> rpm/1
  connections:
  R/RConn1 -- Ideal Rotational Motion Sensor/LConn1
  Mechanical Rotational Reference/LConn1 -- Ideal Rotational Motion Sensor/RConn1
  Ideal Rotational Motion Sensor/RConn2 -- PS-Simulink Converter/LConn1

== system SHEV_EXAMPLE1/MOTOR/RPM SENSOR ==
  Ideal Rotational Motion Sensor : fl_lib/Mechanical/Mechanical Sensors/Ideal Rotational Motion Sensor  reference=foundation.enum.MeasurementReference.difference  acceleration_port=false  velocity_port=true  position_port=true  wrap_angle=false  offset=0 rad
  Mechanical Rotational Reference : fl_lib/Mechanical/Rotational Elements/Mechanical Rotational Reference
  PS-Simulink Converter : nesl_utility/PS-Simulink Converter  PhysicalDomain=network_engine_domain  SubClassName=ps_output  LeftPortType=input  RightPortType=output  PseudoPeriodic=off  Frequencies=[]  VectorFormat=1-D array  Unit=rpm  AffineConversion=off
  R : PMIOPort  Side=Left
  rpm : Outport
  wires:
  PS-Simulink Converter/1 -> rpm/1
  connections:
  R/RConn1 -- Ideal Rotational Motion Sensor/LConn1
  Mechanical Rotational Reference/LConn1 -- Ideal Rotational Motion Sensor/RConn1
  Ideal Rotational Motion Sensor/RConn2 -- PS-Simulink Converter/LConn1

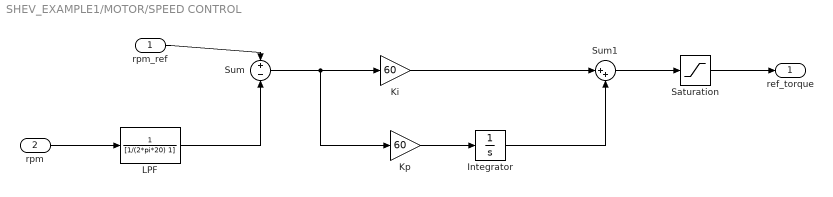
== system SHEV_EXAMPLE1/MOTOR/SPEED CONTROL ==
  rpm_ref : Inport
  rpm : Inport  Port=2
  Integrator : Integrator  LimitOutput=on  UpperSaturationLimit=40  LowerSaturationLimit=-40
  Ki : Gain  Gain=60
  Kp : Gain  Gain=60
  LPF : TransferFcn  Denominator=[1/(2*pi*20) 1]
  Saturation : Saturate  UpperLimit=400  LowerLimit=-400
  Sum : Sum  Inputs=+-
  Sum1 : Sum  Inputs=|++
  ref_torque : Outport
  wires:
  rpm_ref/1 -> Sum/1
  rpm/1 -> LPF/1
  LPF/1 -> Sum/2
  Sum/1 -> Ki/1, Kp/1
  Ki/1 -> Sum1/1
  Kp/1 -> Integrator/1
  Integrator/1 -> Sum1/2
  Sum1/1 -> Saturation/1
  Saturation/1 -> ref_torque/1
